simulink model "week2problem3"  (R2020b)
settings: Solver=VariableStepAuto  StartTime=0.0  StopTime=10.0  RelTol=1e-3
settings Model: Creator=HP  LastModifiedBy=HP

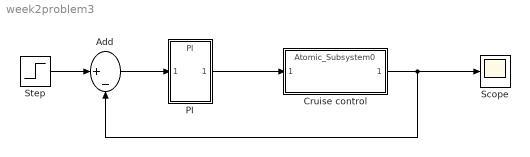
== system week2problem3 ==
  Add : Sum  Inputs=|+-
  "Cruise control " : ModelReference  ModelNameDialog=Atomic_Subsystem0  SimulationMode=Normal  ModelReferenceVersion=1.12
  PI : ModelReference  ModelNameDialog=PI  SimulationMode=Normal  ModelReferenceVersion=1.16
  Scope : Scope
  Step : Step  Time=0  After=5000  SampleTime=0
  wires:
  "Cruise control "/1 -> Add/2, Scope/1
  Step/1 -> Add/1
  Add/1 -> PI/1
  PI/1 -> "Cruise control "/1
